simulink model "building_HVAC_V00_027_AI_2019b"  (R2021b)
settings: Solver=ode3  StartTime=1425600  StopTime=1429297  FixedStep=0.1  RelTol=1e-3
model workspace (MAT data in the model file):
  A = 0
  pystep = 1
values from neighbouring files (symbols this model uses):
  Air_Cp = [1007 1007 1006 1006 1006 1006 1006 1006 1006 1006 1007 1007 ... (21 elements, 21x1)]    [data_07.mat]    (also in data_08.mat)
  Air_density = [1.783 1.582 1.422 1.367 1.341 1.316 1.292 1.268 1.246 1.225 1.204 1.184 ... (32 elements, 32x1)]    [data_07.mat]    (also in data_08.mat)
  Air_dynamic_viscosity_PaS = [1.318e-05 1.456e-05 1.588e-05 1.64e-05 1.665e-05 1.69e-05 1.715e-05 1.74e-05 1.764e-05 1.789e-05 1.813e-05 1.837e-05 ... (32 elements, 32x1)]    [data_07.mat]    (also in data_08.mat)
  Air_enthalpy = [325420 335490 345550 355620 365680 375730 385790 395850 405910 415970 426040 436110 ... (21 elements, 21x1)]    [data_07.mat]    (also in data_08.mat)
  Air_prandtl_number = [0.734 0.72 0.711 0.707 0.705 0.701 0.699 0.698 0.699 0.702]    [data_07.mat]    (also in data_08.mat)
  Air_Temp_for_Cp = [200 210 220 230 240 250 260 270 280 290 300 310 ... (21 elements, 21x1)]    [data_07.mat]    (also in data_08.mat)
  Air_Temp_for_density = [-75 -50 -25 -15 -10 -5 0 5 10 15 20 25 ... (32 elements, 32x1)]    [data_07.mat]    (also in data_08.mat)
  Air_Temp_for_dynamic_viscosity = [-75 -50 -25 -15 -10 -5 0 5 10 15 20 25 ... (32 elements, 32x1)]    [data_07.mat]    (also in data_08.mat)
  Air_Temp_for_enthalpy = [200 210 220 230 240 250 260 270 280 290 300 310 ... (21 elements, 21x1)]    [data_07.mat]    (also in data_08.mat)
  Air_Temp_for_prandtl_number = [-100 -50 0 25 50 100 150 200 250 300]    [data_07.mat]    (also in data_08.mat)
  Air_Temp_for_thermal_conductivity = [-190 -150 -100 -75 -50 -25 -15 -10 -5 0 5 10 ... (35 elements, 35x1)]    [data_07.mat]    (also in data_08.mat)
  Air_thermal_conductivity = [0.00782 0.01169 0.0162 0.01834 0.02041 0.02241 0.0232 0.02359 0.02397 0.02436 0.02474 0.02512 ... (35 elements, 35x1)]    [data_07.mat]    (also in data_08.mat)
  Ambient_Solar_heat_Seoul_20200701_to_20200731 = [0 0 0 0 0 0 2.777777778 38.88888889 72.22222222 97.22222222 333.3333333 263.8888889 ... (745 elements, 745x1)]    [data_07.mat]    (also in data_08.mat)
  Ambient_Solar_heat_Seoul_20200701_to_20210630 = [0 0 0 0 0 2.777777778 38.88888889 72.22222222 97.22222222 333.3333333 263.8888889 152.7777778 ... (8736 elements, 8736x1)]    [data_07.mat]    (also in data_08.mat)
  Ambient_Solar_heat_Seoul_20200801_to_20200831 = [0 0 0 0 0 0 2.777777778 11.11111111 38.88888889 63.88888889 127.7777778 258.3333333 ... (745 elements, 745x1)]    [data_07.mat]    (also in data_08.mat)
  Ambient_Solar_heat_Seoul_20200901_to_20200930 = [0 0 0 0 0 0 0 22.22222222 108.3333333 141.6666667 211.1111111 386.1111111 ... (721 elements, 721x1)]    [data_07.mat]    (also in data_08.mat)
  Ambient_Temp_Seoul_20200701_to_20200731 = [18.8 18.8 18.7 18.4 18.2 18.2 18.3 18.5 19.1 19.6 21.2 21.6 ... (745 elements, 745x1)]    [data_07.mat]    (also in data_08.mat)
  Ambient_Temp_Seoul_20200701_to_20210630 = [18.8 18.7 18.4 18.2 18.2 18.3 18.5 19.1 19.6 21.2 21.6 21.7 ... (8736 elements, 8736x1)]    [data_07.mat]    (also in data_08.mat)
  Ambient_Temp_Seoul_20200801_to_20200831 = [25 24.6 24.6 24.7 24.7 24.5 24.3 24.3 24.6 25 25.7 26.8 ... (745 elements, 745x1)]    [data_07.mat]    (also in data_08.mat)
  Ambient_Temp_Seoul_20200901_to_20200930 = [26.2 25.8 25.5 24.9 24.5 24.3 24 23.9 24.4 24.8 25.7 26.6 ... (721 elements, 721x1)]    [data_07.mat]    (also in data_08.mat)
  Ambient_Time_Seoul_20200701_to_20200731 = [0 3600 7200 10800 14400 18000 21600 25200 28800 32400 36000 39600 ... (745 elements, 745x1)]    [data_07.mat]    (also in data_08.mat)
  Ambient_Time_Seoul_20200701_to_20210630 = [0 3600 7200 10800 14400 18000 21600 25200 28800 32400 36000 39600 ... (8736 elements, 8736x1)]    [data_07.mat]    (also in data_08.mat)
  Ambient_Time_Seoul_20200901_to_20200930 = [0 3600 7200 10800 14400 18000 21600 25200 28800 32400 36000 39600 ... (721 elements, 721x1)]    [data_07.mat]    (also in data_08.mat)
  Ambient_Water_Vapor_Pressure_Seoul_20200701_to_20200731 = [18.4 18.8 18.6 18.2 17.9 17.7 18.6 18.6 18.5 19.1 19.9 19.5 ... (745 elements, 745x1)]    [data_07.mat]    (also in data_08.mat)
  Ambient_Water_Vapor_Pressure_Seoul_20200701_to_20210630 = [18.8 18.6 18.2 17.9 17.7 18.6 18.6 18.5 19.1 19.9 19.5 19.4 ... (8736 elements, 8736x1)]    [data_07.mat]    (also in data_08.mat)
  Ambient_Water_Vapor_Pressure_Seoul_20200801_to_20200831 = [28.4 27.7 28.1 28.8 29.1 28.8 28.8 29.1 29.7 30 31.3 29.8 ... (745 elements, 745x1)]    [data_07.mat]    (also in data_08.mat)
  Ambient_Water_Vapor_Pressure_Seoul_20200901_to_20200930 = [26.1 25.8 25.6 24.7 24 24.3 22.9 23.1 23.1 22.8 24 24.3 ... (721 elements, 721x1)]    [data_07.mat]    (also in data_08.mat)
  Ambient_wind_speed_Seoul_20200701_to_20200731 = [3.7 3 3 2.3 1.2 1.5 3.1 1.4 1 1.4 2.5 2.1 ... (745 elements, 745x1)]    [data_07.mat]    (also in data_08.mat)
  Ambient_wind_speed_Seoul_20200701_to_20210630 = [3 3 2.3 1.2 1.5 3.1 1.4 1 1.4 2.5 2.1 2 ... (8736 elements, 8736x1)]    [data_07.mat]    (also in data_08.mat)
  Ambient_wind_speed_Seoul_20200801_to_20200831 = [3.4 0.5 0.5 1.2 0.8 1.3 1.8 1.4 1.2 1.1 1.8 3.4 ... (745 elements, 745x1)]    [data_07.mat]    (also in data_08.mat)
  Ambient_wind_speed_Seoul_20200901_to_20200930 = [2.3 2.2 2.5 2.6 2.4 2.1 1.7 2.7 2.6 2.5 1.5 1.8 ... (721 elements, 721x1)]    [data_07.mat]    (also in data_08.mat)
  init_time = start_time +60    [SIMULINK_RUn.m]    (also in data_07.mat = 0; data_08.mat = 1425660)
  Initial_Temp = 273 + 28    (= 301)    [SIMULINK_RUn.m]    (also in data_07.mat = 285; data_08.mat = 302)
  Shadow_20200701_to_20210630 = [285 300 315 330 345 360 15 30 45 60 75 90 ... (8736 elements, 8736x1)]    [data_07.mat]    (also in data_08.mat)
  start_time = 12 * 3600 + da * day_to_sec    [SIMULINK_RUn.m]    (also in data_07.mat = 0; data_08.mat = 1425600)
  Under_30cm_ground_Temp_Seoul_20200701_to_20200731 = [22.6 22.6 22.5 22.5 22.4 22.3 22.3 22.2 22.1 22.1 22 22 ... (745 elements, 745x1)]    [data_07.mat]    (also in data_08.mat)
  Under_30cm_ground_Temp_Seoul_20200701_to_20210630 = [22.6 22.5 22.5 22.4 22.3 22.3 22.2 22.1 22.1 22 22 22 ... (8736 elements, 8736x1)]    [data_07.mat]    (also in data_08.mat)
  Under_30cm_ground_Temp_Seoul_20200801_to_20200831 = [25.6 25.6 25.6 25.5 25.5 25.5 25.4 25.4 25.3 25.3 25.3 25.2 ... (745 elements, 745x1)]    [data_07.mat]    (also in data_08.mat)
  Under_30cm_ground_Temp_Seoul_20200901_to_20200930 = [27.4 27.4 27.4 27.4 27.3 27.3 27.3 27.2 27.2 27.1 27 27 ... (721 elements, 721x1)]    [data_07.mat]    (also in data_08.mat)
  water_saturation_enthalpy_latent = [2500899.39 2498955.8 2496540.3 2494128 2491818 2489411 2487006 2484604 2482303 2479905 2477508 2475213 ... (64 elements, 64x1)]    [data_07.mat]    (also in data_08.mat)
  water_saturation_enthalpy_vapor = [2500900 2502500 2504300 2506100 2508000 2509800 2511600 2513400 2515300 2517100 2518900 2520800 ... (64 elements, 64x1)]    [data_07.mat]    (also in data_08.mat)
  water_saturation_pressure = [611.65 650.03 698.46 750.07 805.02 863.5 925.7 991.83 1062.2 1136.8 1216 1300 ... (64 elements, 64x1)]    [data_07.mat]    (also in data_08.mat)
  water_Temp_for_saturation_enthalpy_latent = [273.16 274 275 276 277 278 279 280 281 282 283 284 ... (64 elements, 64x1)]    [data_07.mat]    (also in data_08.mat)
  water_Temp_for_saturation_enthalpy_vapor = [273.16 274 275 276 277 278 279 280 281 282 283 284 ... (64 elements, 64x1)]    [data_07.mat]    (also in data_08.mat)
  water_Temp_for_saturation_pressure = [273.16 274 275 276 277 278 279 280 281 282 283 284 ... (64 elements, 64x1)]    [data_07.mat]    (also in data_08.mat)
undefined symbols (not defined in the file or in its folder): DiscIntNeverNeededParam
libraries: fuzblock x1
(part 3 of 3)

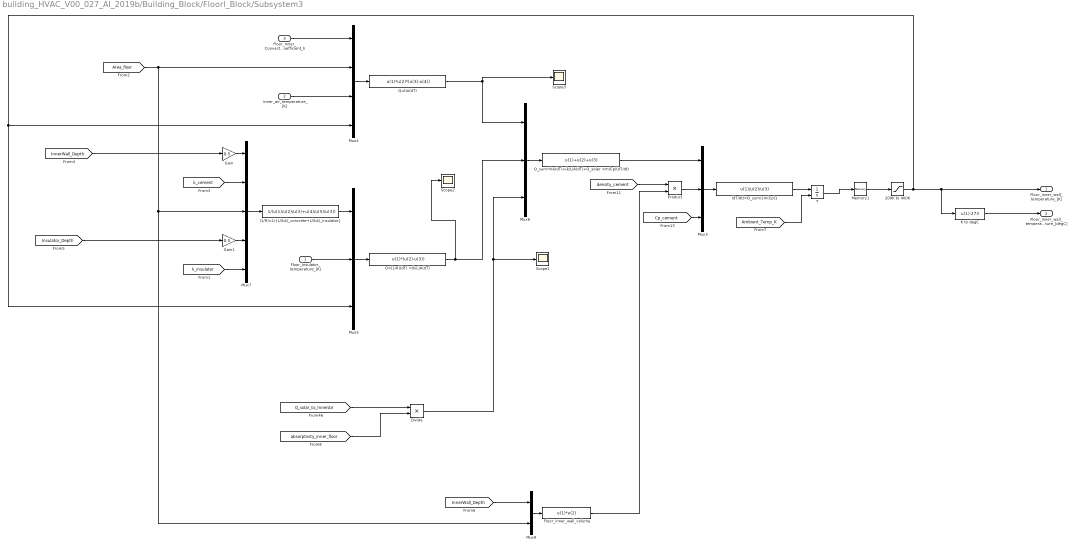
== system building_HVAC_V00_027_AI_2019b/Building_Block/Floorl_Block/Subsystem3 ==
  Floor_Insulator_temperature_[K] : Inport
  Inner_air_temperature_[K] : Inport  Port=2
  Floor_Inner_Convective_coefficient_h : Inport  Port=3
  "(1/R)=1/{L/(kA)_concrete+L/(kA)_insulator}" : Fcn  Expr=1/(u(1)/u(2)/u(3)+u(4)/u(5)/u(3))
  "(dT/dt)=Q_sum/{m(Cp)}" : Fcn  Expr=u(1)/u(2)/u(3)
  200K to 400K : Saturate  UpperLimit=400  LowerLimit=200
  Divide : Product  Inputs=**
  Floor_inner_wall_volume : Fcn  Expr=u(1)*u(2)
  Gain : Gain  Gain=0.5
  Gain1 : Gain  Gain=0.5
  K to degC : Fcn  Expr=u(1)-273
  Memory1 : Memory  InitialCondition=300-5-3  InheritSampleTime=on
  Mux3 : Mux  Inputs=3
  Mux4 : Mux
  Mux5 : Mux  Inputs=3
  Mux6 : Mux  Inputs=3
  Mux7 : Mux  Inputs=5
  Mux9 : Mux  Inputs=2
  Product : Product
  Q=(1/R)(dT) =(k/L)A(dT) : Fcn  Expr=u(1)*(u(2)-u(3))
  Q=hA(dT) : Fcn  Expr=u(1)*u(2)*(u(3)-u(4))
  Q_sum=hA(dT)+(k/L)A(dT)+Q_solar =m(Cp)(dT/dt) : Fcn  Expr=u(1)+u(2)+u(3)
  Scope1 : Scope
  Scope2 : Scope
  Scope3 : Scope
  T : Integrator  InitialConditionSource=external
  Floor_inner_wall_temperature_[K] : Outport
  Floor_inner_wall_temperature_[degC] : Outport  Port=2
  wires:
  K to degC/1 -> Floor_inner_wall_temperature_[degC]/1
  Floor_inner_wall_volume/1 -> Product/2
  [k_insulator] -> Mux7/5
  Gain1/1 -> Mux7/4
  Floor_Insulator_temperature_[K]/1 -> Mux5/2
  Q_sum=hA(dT)+(k/L)A(dT)+Q_solar =m(Cp)(dT/dt)/1 -> Mux3/1
  [k_cement] -> Mux7/2
  Mux7/1 -> "(1/R)=1/{L/(kA)_concrete+L/(kA)_insulator}"/1
  Q=hA(dT)/1 -> Mux6/1, Scope3/1
  "(1/R)=1/{L/(kA)_concrete+L/(kA)_insulator}"/1 -> Mux5/1
  Gain/1 -> Mux7/1
  Memory1/1 -> 200K to 400K/1
  Q=(1/R)(dT) =(k/L)A(dT)/1 -> Scope2/1, Mux6/2
  Mux4/1 -> Q=hA(dT)/1
  Mux5/1 -> Q=(1/R)(dT) =(k/L)A(dT)/1
  200K to 400K/1 -> Mux5/3, Mux4/4, Floor_inner_wall_temperature_[K]/1, K to degC/1
  T/1 -> Memory1/1
  Inner_air_temperature_[K]/1 -> Mux4/3
  [Area_floor] -> Mux9/2, Mux7/3, Mux4/2
  Product/1 -> Mux3/2
  [Cp_cement] -> Mux3/3
  "(dT/dt)=Q_sum/{m(Cp)}"/1 -> T/1
  Mux9/1 -> Floor_inner_wall_volume/1
  [density_cement] -> Product/1
  Mux3/1 -> "(dT/dt)=Q_sum/{m(Cp)}"/1
  Floor_Inner_Convective_coefficient_h/1 -> Mux4/1
  Mux6/1 -> Q_sum=hA(dT)+(k/L)A(dT)+Q_solar =m(Cp)(dT/dt)/1
  [Ambient_Temp_K] -> T/2
  [Q_solar_to_InnerAir] -> Divide/1
  [absorptivity_inner_floor] -> Divide/2
  [InnerWall_Depth] -> Gain/1
  [Insulator_Depth] -> Gain1/1
  Divide/1 -> Scope1/1, Mux6/3
  [InnerWall_Depth] -> Mux9/1

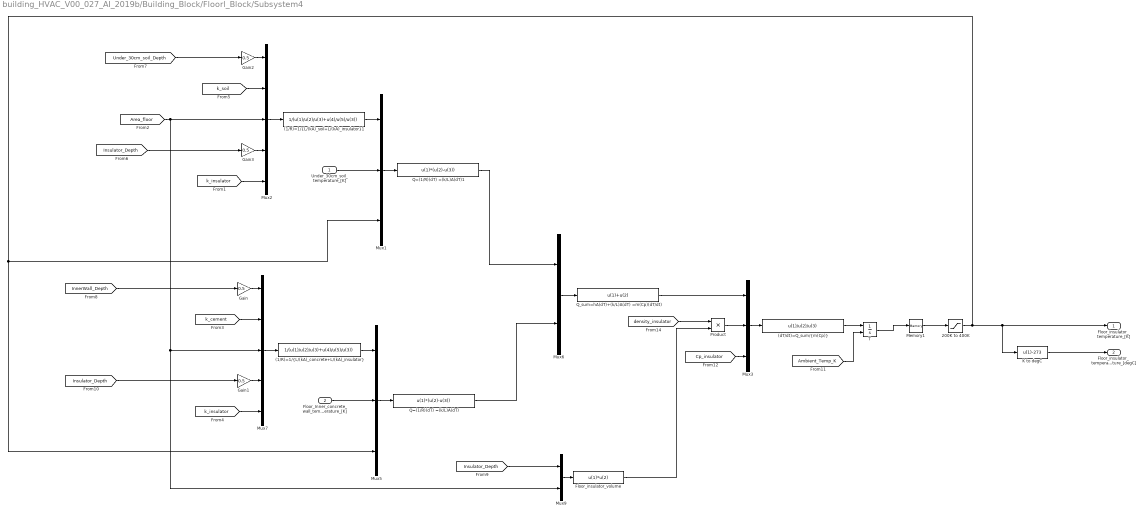
== system building_HVAC_V00_027_AI_2019b/Building_Block/Floorl_Block/Subsystem4 ==
  Under_30cm_soil_temperature_[K] : Inport
  Floor_Inner_concrete_wall_temperature_[K] : Inport  Port=2
  "(1/R)=1/{L/(kA)_concrete+L/(kA)_insulator}" : Fcn  Expr=1/(u(1)/u(2)/u(3)+u(4)/u(5)/u(3))
  "(1/R)=1/{L/(kA)_soil+L/(kA)_insulator}1" : Fcn  Expr=1/(u(1)/u(2)/u(3)+u(4)/u(5)/u(3))
  "(dT/dt)=Q_sum/{m(Cp)}" : Fcn  Expr=u(1)/u(2)/u(3)
  200K to 400K : Saturate  UpperLimit=400  LowerLimit=200
  Floor_insulator_volume : Fcn  Expr=u(1)*u(2)
  Gain{,1..3} (4 alike) : Gain  Gain=0.5
  K to degC : Fcn  Expr=u(1)-273
  Memory1 : Memory  InitialCondition=300  InheritSampleTime=on
  Mux1 : Mux  Inputs=3
  Mux2 : Mux  Inputs=5
  Mux3 : Mux  Inputs=3
  Mux5 : Mux  Inputs=3
  Mux6 : Mux  Inputs=2
  Mux7 : Mux  Inputs=5
  Mux9 : Mux  Inputs=2
  Product : Product
  Q=(1/R)(dT) =(k/L)A(dT) : Fcn  Expr=u(1)*(u(2)-u(3))
  Q=(1/R)(dT) =(k/L)A(dT)1 : Fcn  Expr=u(1)*(u(2)-u(3))
  Q_sum=hA(dT)+(k/L)A(dT) =m(Cp)(dT/dt) : Fcn  Expr=u(1)+u(2)
  T : Integrator  InitialConditionSource=external
  Floor_insulator_temperature_[K] : Outport
  Floor_insulator_temperature_[degC] : Outport  Port=2
  wires:
  Mux6/1 -> Q_sum=hA(dT)+(k/L)A(dT) =m(Cp)(dT/dt)/1
  Mux3/1 -> "(dT/dt)=Q_sum/{m(Cp)}"/1
  [density_insulator] -> Product/1
  Mux9/1 -> Floor_insulator_volume/1
  "(dT/dt)=Q_sum/{m(Cp)}"/1 -> T/1
  [Cp_insulator] -> Mux3/3
  Product/1 -> Mux3/2
  [Area_floor] -> Mux9/2, Mux7/3, Mux2/3
  T/1 -> Memory1/1
  200K to 400K/1 -> K to degC/1, Floor_insulator_temperature_[K]/1, Mux1/3, Mux5/3
  Mux5/1 -> Q=(1/R)(dT) =(k/L)A(dT)/1
  Q=(1/R)(dT) =(k/L)A(dT)/1 -> Mux6/2
  Memory1/1 -> 200K to 400K/1
  Gain/1 -> Mux7/1
  "(1/R)=1/{L/(kA)_concrete+L/(kA)_insulator}"/1 -> Mux5/1
  Q=(1/R)(dT) =(k/L)A(dT)1/1 -> Mux6/1
  Mux7/1 -> "(1/R)=1/{L/(kA)_concrete+L/(kA)_insulator}"/1
  [k_cement] -> Mux7/2
  Q_sum=hA(dT)+(k/L)A(dT) =m(Cp)(dT/dt)/1 -> Mux3/1
  Floor_Inner_concrete_wall_temperature_[K]/1 -> Mux5/2
  Gain1/1 -> Mux7/4
  [k_insulator] -> Mux7/5
  Floor_insulator_volume/1 -> Product/2
  K to degC/1 -> Floor_insulator_temperature_[degC]/1
  [k_insulator] -> Mux2/5
  "(1/R)=1/{L/(kA)_soil+L/(kA)_insulator}1"/1 -> Mux1/1
  Gain2/1 -> Mux2/1
  [k_soil] -> Mux2/2
  Mux1/1 -> Q=(1/R)(dT) =(k/L)A(dT)1/1
  Under_30cm_soil_temperature_[K]/1 -> Mux1/2
  Mux2/1 -> "(1/R)=1/{L/(kA)_soil+L/(kA)_insulator}1"/1
  Gain3/1 -> Mux2/4
  [Ambient_Temp_K] -> T/2
  [Under_30cm_soil_Depth] -> Gain2/1
  [Insulator_Depth] -> Gain3/1
  [InnerWall_Depth] -> Gain/1
  [Insulator_Depth] -> Gain1/1
  [Insulator_Depth] -> Mux9/1

== system building_HVAC_V00_027_AI_2019b/Building_Block/North_Wall_Block/Subsystem1 ==
  North_inner_concrete_wall_temperature_[K] : Inport
  Inner_air_temperature_[K] : Inport  Port=2
  North_Inner_Convective_coefficient_h : Inport  Port=3
  -1000000 to 1000000 : Saturate  UpperLimit=1000000  LowerLimit=-1000000
  Memory : Memory  InheritSampleTime=on
  Mux4 : Mux
  Q=hA(dT) : Fcn  Expr=u(1)*u(2)*(u(3)-u(4))
  Q_North_InnerWall_to_InnerAir_[W] : Outport
  wires:
  Memory/1 -> -1000000 to 1000000/1
  Q=hA(dT)/1 -> Memory/1
  Mux4/1 -> Q=hA(dT)/1
  -1000000 to 1000000/1 -> Q_North_InnerWall_to_InnerAir_[W]/1
  North_inner_concrete_wall_temperature_[K]/1 -> Mux4/3
  [Area_North] -> Mux4/2
  North_Inner_Convective_coefficient_h/1 -> Mux4/1
  Inner_air_temperature_[K]/1 -> Mux4/4

== system building_HVAC_V00_027_AI_2019b/Building_Block/North_Wall_Block/Subsystem2 ==
  Ambient_temperature_[K] : Inport
  North_Insulator_temperature_[K] : Inport  Port=2
  North_Out_Convective_coefficient_h : Inport  Port=3
  "(1/R)=1/{L/(kA)_concrete+L/(kA)_insulator}" : Fcn  Expr=1/(u(1)/u(2)/u(3)+u(4)/u(5)/u(3))
  "(dT/dt)=Q_sum/{m(Cp)}" : Fcn  Expr=u(1)/u(2)/u(3)
  200K to 800K : Saturate  UpperLimit=800  LowerLimit=200
  Divide : Product  Inputs=***
  Gain : Gain  Gain=0.5
  Gain1 : Gain  Gain=0.5
  K to degC : Fcn  Expr=u(1)-273
  Memory1 : Memory  InitialCondition=300  InheritSampleTime=on
  Mux3 : Mux  Inputs=3
  Mux4 : Mux
  Mux5 : Mux  Inputs=3
  Mux6 : Mux  Inputs=3
  Mux7 : Mux  Inputs=5
  Mux9 : Mux  Inputs=2
  North_wall_volume : Fcn  Expr=u(1)*u(2)
  Product : Product
  Q=(1/R)(dT) =(k/L)A(dT) : Fcn  Expr=u(1)*(u(2)-u(3))
  Q=hA(dT) : Fcn  Expr=u(1)*u(2)*(u(3)-u(4))
  Q_sum=hA(dT)+(k/L)A(dT)+Q_solar =m(Cp)(dT/dt) : Fcn  Expr=u(1)+u(2)+u(3)
  T : Integrator  InitialConditionSource=external
  North_outer_concrete_wall_temperature_[K] : Outport
  North_outer_concrete_wall_temperature_[degC] : Outport  Port=2
  wires:
  [absoptivity_wall] -> Divide/2
  [solar_heat_flux] -> Divide/3
  Divide/1 -> Mux6/3
  [Area_North] -> Mux4/2, Mux7/3, Divide/1, Mux9/2
  K to degC/1 -> North_outer_concrete_wall_temperature_[degC]/1
  North_wall_volume/1 -> Product/2
  [k_insulator] -> Mux7/5
  Gain1/1 -> Mux7/4
  North_Insulator_temperature_[K]/1 -> Mux5/2
  Q_sum=hA(dT)+(k/L)A(dT)+Q_solar =m(Cp)(dT/dt)/1 -> Mux3/1
  [k_cement] -> Mux7/2
  Mux7/1 -> "(1/R)=1/{L/(kA)_concrete+L/(kA)_insulator}"/1
  Q=hA(dT)/1 -> Mux6/1
  "(1/R)=1/{L/(kA)_concrete+L/(kA)_insulator}"/1 -> Mux5/1
  Gain/1 -> Mux7/1
  [Insulator_Depth] -> Gain1/1
  Memory1/1 -> 200K to 800K/1
  Q=(1/R)(dT) =(k/L)A(dT)/1 -> Mux6/2
  Mux4/1 -> Q=hA(dT)/1
  Mux5/1 -> Q=(1/R)(dT) =(k/L)A(dT)/1
  200K to 800K/1 -> Mux5/3, Mux4/4, North_outer_concrete_wall_temperature_[K]/1, K to degC/1
  T/1 -> Memory1/1
  [OuterWall_Depth] -> Gain/1
  Ambient_temperature_[K]/1 -> Mux4/3
  [OuterWall_Depth] -> Mux9/1
  Product/1 -> Mux3/2
  [Cp_cement] -> Mux3/3
  "(dT/dt)=Q_sum/{m(Cp)}"/1 -> T/1
  Mux9/1 -> North_wall_volume/1
  [density_cement] -> Product/1
  Mux3/1 -> "(dT/dt)=Q_sum/{m(Cp)}"/1
  North_Out_Convective_coefficient_h/1 -> Mux4/1
  Mux6/1 -> Q_sum=hA(dT)+(k/L)A(dT)+Q_solar =m(Cp)(dT/dt)/1
  [Ambient_Temp_K] -> T/2

== system building_HVAC_V00_027_AI_2019b/Building_Block/North_Wall_Block/Subsystem3 ==
  North_Insulator_temperature_[K] : Inport
  Inner_air_temperature_[K] : Inport  Port=2
  North_Inner_Convective_coefficient_h : Inport  Port=3
  "(1/R)=1/{L/(kA)_concrete+L/(kA)_insulator}" : Fcn  Expr=1/(u(1)/u(2)/u(3)+u(4)/u(5)/u(3))
  "(dT/dt)=Q_sum/{m(Cp)}" : Fcn  Expr=u(1)/u(2)/u(3)
  200K to 400K : Saturate  UpperLimit=400  LowerLimit=200
  Divide : Product  Inputs=**
  Gain : Gain  Gain=0.5
  Gain1 : Gain  Gain=0.5
  K to degC : Fcn  Expr=u(1)-273
  Memory1 : Memory  InitialCondition=300  InheritSampleTime=on
  Mux3 : Mux  Inputs=3
  Mux4 : Mux
  Mux5 : Mux  Inputs=3
  Mux6 : Mux  Inputs=3
  Mux7 : Mux  Inputs=5
  Mux9 : Mux  Inputs=2
  North_wall_volume : Fcn  Expr=u(1)*u(2)
  Product : Product
  Q=(1/R)(dT) =(k/L)A(dT) : Fcn  Expr=u(1)*(u(2)-u(3))
  Q=hA(dT) : Fcn  Expr=u(1)*u(2)*(u(3)-u(4))
  Q_sum=hA(dT)+(k/L)A(dT)+Q_solar =m(Cp)(dT/dt) : Fcn  Expr=u(1)+u(2)
  T : Integrator  InitialConditionSource=external
  North_inner_concrete_wall_temperature_[K] : Outport
  North_inner_concrete_wall_temperature_[degC] : Outport  Port=2
  wires:
  Mux6/1 -> Q_sum=hA(dT)+(k/L)A(dT)+Q_solar =m(Cp)(dT/dt)/1
  North_Inner_Convective_coefficient_h/1 -> Mux4/1
  Mux3/1 -> "(dT/dt)=Q_sum/{m(Cp)}"/1
  [density_cement] -> Product/1
  Mux9/1 -> North_wall_volume/1
  "(dT/dt)=Q_sum/{m(Cp)}"/1 -> T/1
  [Cp_cement] -> Mux3/3
  Product/1 -> Mux3/2
  [InnerWall_Depth] -> Mux9/1
  [Area_North] -> Mux4/2, Mux7/3, Mux9/2
  Inner_air_temperature_[K]/1 -> Mux4/3
  [InnerWall_Depth] -> Gain/1
  T/1 -> Memory1/1
  200K to 400K/1 -> K to degC/1, North_inner_concrete_wall_temperature_[K]/1, Mux4/4, Mux5/3
  Mux5/1 -> Q=(1/R)(dT) =(k/L)A(dT)/1
  Mux4/1 -> Q=hA(dT)/1
  Q=(1/R)(dT) =(k/L)A(dT)/1 -> Mux6/2
  Memory1/1 -> 200K to 400K/1
  [Insulator_Depth] -> Gain1/1
  Gain/1 -> Mux7/1
  "(1/R)=1/{L/(kA)_concrete+L/(kA)_insulator}"/1 -> Mux5/1
  Q=hA(dT)/1 -> Mux6/1
  Mux7/1 -> "(1/R)=1/{L/(kA)_concrete+L/(kA)_insulator}"/1
  [k_cement] -> Mux7/2
  Q_sum=hA(dT)+(k/L)A(dT)+Q_solar =m(Cp)(dT/dt)/1 -> Mux3/1
  North_Insulator_temperature_[K]/1 -> Mux5/2
  Gain1/1 -> Mux7/4
  [k_insulator] -> Mux7/5
  North_wall_volume/1 -> Product/2
  K to degC/1 -> North_inner_concrete_wall_temperature_[degC]/1
  [Ambient_Temp_K] -> T/2
  [absorptivity_inner_wall_North] -> Divide/2
  [Q_solar_to_InnerAir] -> Divide/1
  Divide/1 -> Mux6/3

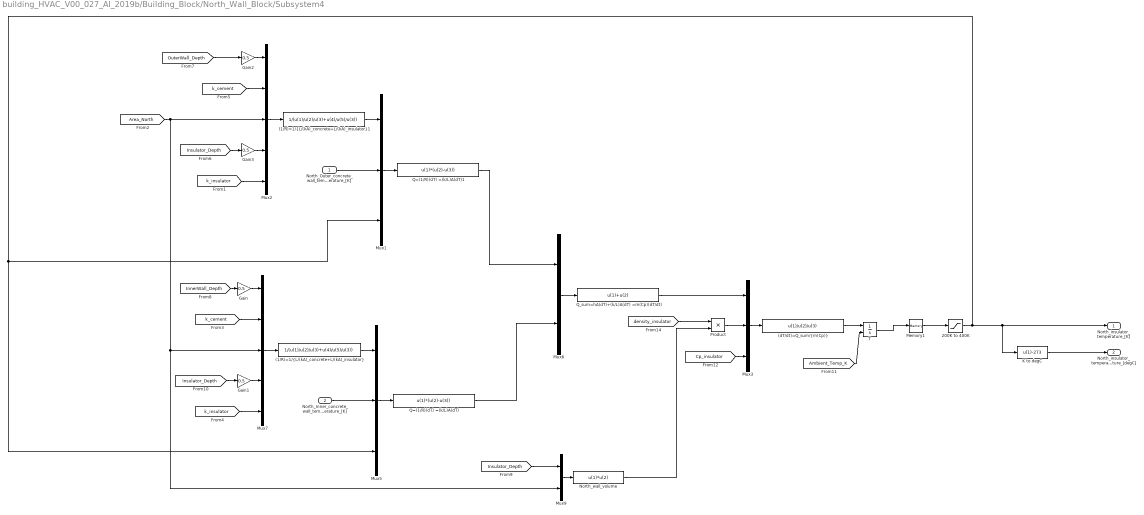
== system building_HVAC_V00_027_AI_2019b/Building_Block/North_Wall_Block/Subsystem4 ==
  North_Outer_concrete_wall_temperature_[K] : Inport
  North_Inner_concrete_wall_temperature_[K] : Inport  Port=2
  "(1/R)=1/{L/(kA)_concrete+L/(kA)_insulator}" : Fcn  Expr=1/(u(1)/u(2)/u(3)+u(4)/u(5)/u(3))
  "(1/R)=1/{L/(kA)_concrete+L/(kA)_insulator}1" : Fcn  Expr=1/(u(1)/u(2)/u(3)+u(4)/u(5)/u(3))
  "(dT/dt)=Q_sum/{m(Cp)}" : Fcn  Expr=u(1)/u(2)/u(3)
  200K to 400K : Saturate  UpperLimit=400  LowerLimit=200
  Gain{,1..3} (4 alike) : Gain  Gain=0.5
  K to degC : Fcn  Expr=u(1)-273
  Memory1 : Memory  InitialCondition=300  InheritSampleTime=on
  Mux1 : Mux  Inputs=3
  Mux2 : Mux  Inputs=5
  Mux3 : Mux  Inputs=3
  Mux5 : Mux  Inputs=3
  Mux6 : Mux  Inputs=2
  Mux7 : Mux  Inputs=5
  Mux9 : Mux  Inputs=2
  North_wall_volume : Fcn  Expr=u(1)*u(2)
  Product : Product
  Q=(1/R)(dT) =(k/L)A(dT) : Fcn  Expr=u(1)*(u(2)-u(3))
  Q=(1/R)(dT) =(k/L)A(dT)1 : Fcn  Expr=u(1)*(u(2)-u(3))
  Q_sum=hA(dT)+(k/L)A(dT) =m(Cp)(dT/dt) : Fcn  Expr=u(1)+u(2)
  T : Integrator  InitialConditionSource=external
  North_insulator_temperature_[K] : Outport
  North_insulator_temperature_[degC] : Outport  Port=2
  wires:
  [OuterWall_Depth] -> Gain2/1
  Gain3/1 -> Mux2/4
  Mux2/1 -> "(1/R)=1/{L/(kA)_concrete+L/(kA)_insulator}1"/1
  North_Outer_concrete_wall_temperature_[K]/1 -> Mux1/2
  Mux1/1 -> Q=(1/R)(dT) =(k/L)A(dT)1/1
  [Insulator_Depth] -> Gain3/1
  [k_cement] -> Mux2/2
  Gain2/1 -> Mux2/1
  "(1/R)=1/{L/(kA)_concrete+L/(kA)_insulator}1"/1 -> Mux1/1
  [k_insulator] -> Mux2/5
  K to degC/1 -> North_insulator_temperature_[degC]/1
  North_wall_volume/1 -> Product/2
  [k_insulator] -> Mux7/5
  Gain1/1 -> Mux7/4
  North_Inner_concrete_wall_temperature_[K]/1 -> Mux5/2
  Q_sum=hA(dT)+(k/L)A(dT) =m(Cp)(dT/dt)/1 -> Mux3/1
  [k_cement] -> Mux7/2
  Mux7/1 -> "(1/R)=1/{L/(kA)_concrete+L/(kA)_insulator}"/1
  Q=(1/R)(dT) =(k/L)A(dT)1/1 -> Mux6/1
  "(1/R)=1/{L/(kA)_concrete+L/(kA)_insulator}"/1 -> Mux5/1
  Gain/1 -> Mux7/1
  [Insulator_Depth] -> Gain1/1
  Memory1/1 -> 200K to 400K/1
  Q=(1/R)(dT) =(k/L)A(dT)/1 -> Mux6/2
  Mux5/1 -> Q=(1/R)(dT) =(k/L)A(dT)/1
  200K to 400K/1 -> Mux5/3, Mux1/3, North_insulator_temperature_[K]/1, K to degC/1
  T/1 -> Memory1/1
  [InnerWall_Depth] -> Gain/1
  [Area_North] -> Mux2/3, Mux7/3, Mux9/2
  [Insulator_Depth] -> Mux9/1
  Product/1 -> Mux3/2
  [Cp_insulator] -> Mux3/3
  "(dT/dt)=Q_sum/{m(Cp)}"/1 -> T/1
  Mux9/1 -> North_wall_volume/1
  [density_insulator] -> Product/1
  Mux3/1 -> "(dT/dt)=Q_sum/{m(Cp)}"/1
  Mux6/1 -> Q_sum=hA(dT)+(k/L)A(dT) =m(Cp)(dT/dt)/1
  [Ambient_Temp_K] -> T/2

== system building_HVAC_V00_027_AI_2019b/Building_Block/South_Wall_Block/Subsystem1 ==
  South_inner_concrete_wall_temperature_[K] : Inport
  Inner_air_temperature_[K] : Inport  Port=2
  South_Inner_Convective_coefficient_h : Inport  Port=3
  -1000000 to 1000000 : Saturate  UpperLimit=1000000  LowerLimit=-1000000
  Memory : Memory  InheritSampleTime=on
  Mux4 : Mux
  Q=hA(dT) : Fcn  Expr=u(1)*u(2)*(u(3)-u(4))
  Q_South_InnerWall_to_InnerAir_[W] : Outport
  wires:
  South_Inner_Convective_coefficient_h/1 -> Mux4/1
  [Area_South] -> Mux4/2
  -1000000 to 1000000/1 -> Q_South_InnerWall_to_InnerAir_[W]/1
  Mux4/1 -> Q=hA(dT)/1
  Q=hA(dT)/1 -> Memory/1
  Memory/1 -> -1000000 to 1000000/1
  South_inner_concrete_wall_temperature_[K]/1 -> Mux4/3
  Inner_air_temperature_[K]/1 -> Mux4/4

== system building_HVAC_V00_027_AI_2019b/Building_Block/South_Wall_Block/Subsystem2 ==
  Ambient_temperature_[K] : Inport
  South_Insulator_temperature_[K] : Inport  Port=2
  South_Out_Convective_coefficient_h : Inport  Port=3
  "(1/R)=1/{L/(kA)_concrete+L/(kA)_insulator}" : Fcn  Expr=1/(u(1)/u(2)/u(3)+u(4)/u(5)/u(3))
  "(dT/dt)=Q_sum/{m(Cp)}" : Fcn  Expr=u(1)/u(2)/u(3)
  200K to 800K : Saturate  UpperLimit=800  LowerLimit=200
  Divide : Product  Inputs=***
  Gain : Gain  Gain=0.5
  Gain1 : Gain  Gain=0.5
  K to degC : Fcn  Expr=u(1)-273
  Memory1 : Memory  InitialCondition=300  InheritSampleTime=on
  Mux3 : Mux  Inputs=3
  Mux4 : Mux
  Mux5 : Mux  Inputs=3
  Mux6 : Mux  Inputs=3
  Mux7 : Mux  Inputs=5
  Mux9 : Mux  Inputs=2
  Product : Product
  Q=(1/R)(dT) =(k/L)A(dT) : Fcn  Expr=u(1)*(u(2)-u(3))
  Q=hA(dT) : Fcn  Expr=u(1)*u(2)*(u(3)-u(4))
  Q_sum=hA(dT)+(k/L)A(dT)+Q_solar =m(Cp)(dT/dt) : Fcn  Expr=u(1)+u(2)+u(3)
  South_wall_volume : Fcn  Expr=u(1)*u(2)
  T : Integrator  InitialConditionSource=external
  South_outer_concrete_wall_temperature_[K] : Outport
  South_outer_concrete_wall_temperature_[degC] : Outport  Port=2
  wires:
  Mux6/1 -> Q_sum=hA(dT)+(k/L)A(dT)+Q_solar =m(Cp)(dT/dt)/1
  South_Out_Convective_coefficient_h/1 -> Mux4/1
  Mux3/1 -> "(dT/dt)=Q_sum/{m(Cp)}"/1
  [density_cement] -> Product/1
  Mux9/1 -> South_wall_volume/1
  "(dT/dt)=Q_sum/{m(Cp)}"/1 -> T/1
  [Cp_cement] -> Mux3/3
  Product/1 -> Mux3/2
  [OuterWall_Depth] -> Mux9/1
  Ambient_temperature_[K]/1 -> Mux4/3
  [OuterWall_Depth] -> Gain/1
  T/1 -> Memory1/1
  200K to 800K/1 -> K to degC/1, South_outer_concrete_wall_temperature_[K]/1, Mux4/4, Mux5/3
  Mux5/1 -> Q=(1/R)(dT) =(k/L)A(dT)/1
  Mux4/1 -> Q=hA(dT)/1
  Q=(1/R)(dT) =(k/L)A(dT)/1 -> Mux6/2
  Memory1/1 -> 200K to 800K/1
  [Insulator_Depth] -> Gain1/1
  Gain/1 -> Mux7/1
  "(1/R)=1/{L/(kA)_concrete+L/(kA)_insulator}"/1 -> Mux5/1
  Q=hA(dT)/1 -> Mux6/1
  Mux7/1 -> "(1/R)=1/{L/(kA)_concrete+L/(kA)_insulator}"/1
  [k_cement] -> Mux7/2
  Q_sum=hA(dT)+(k/L)A(dT)+Q_solar =m(Cp)(dT/dt)/1 -> Mux3/1
  South_Insulator_temperature_[K]/1 -> Mux5/2
  Gain1/1 -> Mux7/4
  [k_insulator] -> Mux7/5
  South_wall_volume/1 -> Product/2
  K to degC/1 -> South_outer_concrete_wall_temperature_[degC]/1
  [Area_South] -> Mux9/2, Divide/1, Mux7/3, Mux4/2
  Divide/1 -> Mux6/3
  [solar_heat_flux] -> Divide/3
  [absoptivity_wall] -> Divide/2
  [Ambient_Temp_K] -> T/2

== system building_HVAC_V00_027_AI_2019b/Building_Block/South_Wall_Block/Subsystem3 ==
  South_Insulator_temperature_[K] : Inport
  Inner_air_temperature_[K] : Inport  Port=2
  South_Inner_Convective_coefficient_h : Inport  Port=3
  "(1/R)=1/{L/(kA)_concrete+L/(kA)_insulator}" : Fcn  Expr=1/(u(1)/u(2)/u(3)+u(4)/u(5)/u(3))
  "(dT/dt)=Q_sum/{m(Cp)}" : Fcn  Expr=u(1)/u(2)/u(3)
  200K to 400K : Saturate  UpperLimit=400  LowerLimit=200
  Divide : Product  Inputs=**
  Gain : Gain  Gain=0.5
  Gain1 : Gain  Gain=0.5
  K to degC : Fcn  Expr=u(1)-273
  Memory1 : Memory  InitialCondition=300  InheritSampleTime=on
  Mux3 : Mux  Inputs=3
  Mux4 : Mux
  Mux5 : Mux  Inputs=3
  Mux6 : Mux  Inputs=3
  Mux7 : Mux  Inputs=5
  Mux9 : Mux  Inputs=2
  Product : Product
  Q=(1/R)(dT) =(k/L)A(dT) : Fcn  Expr=u(1)*(u(2)-u(3))
  Q=hA(dT) : Fcn  Expr=u(1)*u(2)*(u(3)-u(4))
  Q_sum=hA(dT)+(k/L)A(dT)_Q_solar =m(Cp)(dT/dt) : Fcn  Expr=u(1)+u(2)
  South_wall_volume : Fcn  Expr=u(1)*u(2)
  T : Integrator  InitialConditionSource=external
  South_inner_concrete_wall_temperature_[K] : Outport
  South_inner_concrete_wall_temperature_[degC] : Outport  Port=2
  wires:
  K to degC/1 -> South_inner_concrete_wall_temperature_[degC]/1
  South_wall_volume/1 -> Product/2
  [k_insulator] -> Mux7/5
  Gain1/1 -> Mux7/4
  South_Insulator_temperature_[K]/1 -> Mux5/2
  Q_sum=hA(dT)+(k/L)A(dT)_Q_solar =m(Cp)(dT/dt)/1 -> Mux3/1
  [k_cement] -> Mux7/2
  Mux7/1 -> "(1/R)=1/{L/(kA)_concrete+L/(kA)_insulator}"/1
  Q=hA(dT)/1 -> Mux6/1
  "(1/R)=1/{L/(kA)_concrete+L/(kA)_insulator}"/1 -> Mux5/1
  Gain/1 -> Mux7/1
  [Insulator_Depth] -> Gain1/1
  Memory1/1 -> 200K to 400K/1
  Q=(1/R)(dT) =(k/L)A(dT)/1 -> Mux6/2
  Mux4/1 -> Q=hA(dT)/1
  Mux5/1 -> Q=(1/R)(dT) =(k/L)A(dT)/1
  200K to 400K/1 -> Mux5/3, Mux4/4, South_inner_concrete_wall_temperature_[K]/1, K to degC/1
  T/1 -> Memory1/1
  [InnerWall_Depth] -> Gain/1
  Inner_air_temperature_[K]/1 -> Mux4/3
  [Area_South] -> Mux9/2, Mux7/3, Mux4/2
  [InnerWall_Depth] -> Mux9/1
  Product/1 -> Mux3/2
  [Cp_cement] -> Mux3/3
  "(dT/dt)=Q_sum/{m(Cp)}"/1 -> T/1
  Mux9/1 -> South_wall_volume/1
  [density_cement] -> Product/1
  Mux3/1 -> "(dT/dt)=Q_sum/{m(Cp)}"/1
  South_Inner_Convective_coefficient_h/1 -> Mux4/1
  Mux6/1 -> Q_sum=hA(dT)+(k/L)A(dT)_Q_solar =m(Cp)(dT/dt)/1
  [Ambient_Temp_K] -> T/2
  Divide/1 -> Mux6/3
  [Q_solar_to_InnerAir] -> Divide/1
  [absorptivity_inner_wall_South] -> Divide/2

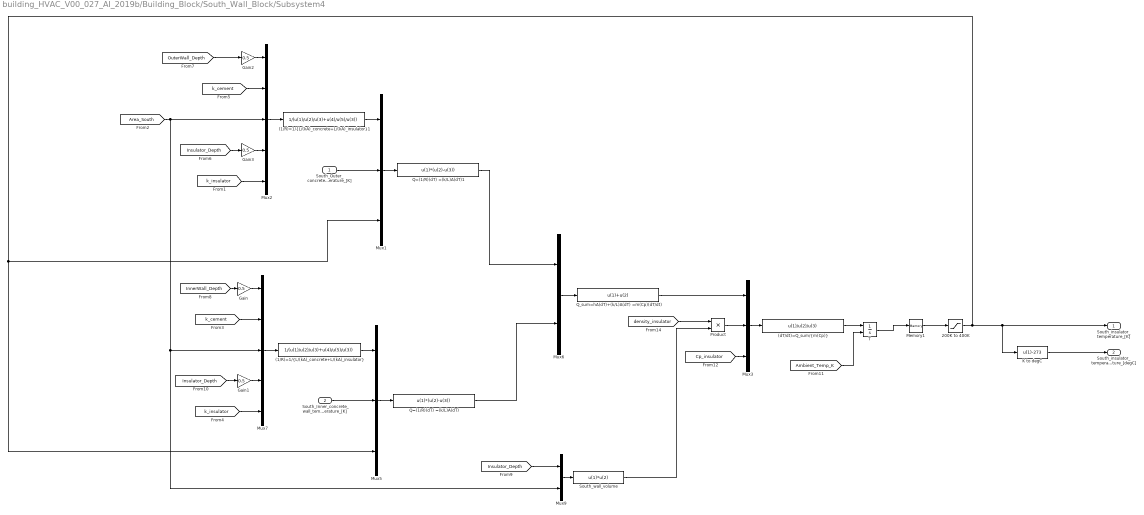
== system building_HVAC_V00_027_AI_2019b/Building_Block/South_Wall_Block/Subsystem4 ==
  South_Outer_concrete_wall_temperature_[K] : Inport
  South_Inner_concrete_wall_temperature_[K] : Inport  Port=2
  "(1/R)=1/{L/(kA)_concrete+L/(kA)_insulator}" : Fcn  Expr=1/(u(1)/u(2)/u(3)+u(4)/u(5)/u(3))
  "(1/R)=1/{L/(kA)_concrete+L/(kA)_insulator}1" : Fcn  Expr=1/(u(1)/u(2)/u(3)+u(4)/u(5)/u(3))
  "(dT/dt)=Q_sum/{m(Cp)}" : Fcn  Expr=u(1)/u(2)/u(3)
  200K to 400K : Saturate  UpperLimit=400  LowerLimit=200
  Gain{,1..3} (4 alike) : Gain  Gain=0.5
  K to degC : Fcn  Expr=u(1)-273
  Memory1 : Memory  InitialCondition=300  InheritSampleTime=on
  Mux1 : Mux  Inputs=3
  Mux2 : Mux  Inputs=5
  Mux3 : Mux  Inputs=3
  Mux5 : Mux  Inputs=3
  Mux6 : Mux  Inputs=2
  Mux7 : Mux  Inputs=5
  Mux9 : Mux  Inputs=2
  Product : Product
  Q=(1/R)(dT) =(k/L)A(dT) : Fcn  Expr=u(1)*(u(2)-u(3))
  Q=(1/R)(dT) =(k/L)A(dT)1 : Fcn  Expr=u(1)*(u(2)-u(3))
  Q_sum=hA(dT)+(k/L)A(dT) =m(Cp)(dT/dt) : Fcn  Expr=u(1)+u(2)
  South_wall_volume : Fcn  Expr=u(1)*u(2)
  T : Integrator  InitialConditionSource=external
  South_insulator_temperature_[K] : Outport
  South_insulator_temperature_[degC] : Outport  Port=2
  wires:
  Mux6/1 -> Q_sum=hA(dT)+(k/L)A(dT) =m(Cp)(dT/dt)/1
  Mux3/1 -> "(dT/dt)=Q_sum/{m(Cp)}"/1
  [density_insulator] -> Product/1
  Mux9/1 -> South_wall_volume/1
  "(dT/dt)=Q_sum/{m(Cp)}"/1 -> T/1
  [Cp_insulator] -> Mux3/3
  Product/1 -> Mux3/2
  [Insulator_Depth] -> Mux9/1
  [Area_South] -> Mux9/2, Mux7/3, Mux2/3
  [InnerWall_Depth] -> Gain/1
  T/1 -> Memory1/1
  200K to 400K/1 -> K to degC/1, South_insulator_temperature_[K]/1, Mux1/3, Mux5/3
  Mux5/1 -> Q=(1/R)(dT) =(k/L)A(dT)/1
  Q=(1/R)(dT) =(k/L)A(dT)/1 -> Mux6/2
  Memory1/1 -> 200K to 400K/1
  [Insulator_Depth] -> Gain1/1
  Gain/1 -> Mux7/1
  "(1/R)=1/{L/(kA)_concrete+L/(kA)_insulator}"/1 -> Mux5/1
  Q=(1/R)(dT) =(k/L)A(dT)1/1 -> Mux6/1
  Mux7/1 -> "(1/R)=1/{L/(kA)_concrete+L/(kA)_insulator}"/1
  [k_cement] -> Mux7/2
  Q_sum=hA(dT)+(k/L)A(dT) =m(Cp)(dT/dt)/1 -> Mux3/1
  South_Inner_concrete_wall_temperature_[K]/1 -> Mux5/2
  Gain1/1 -> Mux7/4
  [k_insulator] -> Mux7/5
  South_wall_volume/1 -> Product/2
  K to degC/1 -> South_insulator_temperature_[degC]/1
  [k_insulator] -> Mux2/5
  "(1/R)=1/{L/(kA)_concrete+L/(kA)_insulator}1"/1 -> Mux1/1
  Gain2/1 -> Mux2/1
  [k_cement] -> Mux2/2
  [Insulator_Depth] -> Gain3/1
  Mux1/1 -> Q=(1/R)(dT) =(k/L)A(dT)1/1
  South_Outer_concrete_wall_temperature_[K]/1 -> Mux1/2
  Mux2/1 -> "(1/R)=1/{L/(kA)_concrete+L/(kA)_insulator}1"/1
  Gain3/1 -> Mux2/4
  [OuterWall_Depth] -> Gain2/1
  [Ambient_Temp_K] -> T/2

== system building_HVAC_V00_027_AI_2019b/Building_Block/West_Wall_Block/Subsystem1 ==
  West_inner_concrete_wall_temperature_[K] : Inport
  Inner_air_temperature_[K] : Inport  Port=2
  West_Inner_Convective_coefficient_h : Inport  Port=3
  -1000000 to 1000000 : Saturate  UpperLimit=1000000  LowerLimit=-1000000
  Memory : Memory  InheritSampleTime=on
  Mux4 : Mux
  Q=hA(dT) : Fcn  Expr=u(1)*u(2)*(u(3)-u(4))
  Q_West_InnerWall_to_InnerAir_[W] : Outport
  wires:
  West_Inner_Convective_coefficient_h/1 -> Mux4/1
  [Area_West] -> Mux4/2
  West_inner_concrete_wall_temperature_[K]/1 -> Mux4/3
  -1000000 to 1000000/1 -> Q_West_InnerWall_to_InnerAir_[W]/1
  Mux4/1 -> Q=hA(dT)/1
  Q=hA(dT)/1 -> Memory/1
  Memory/1 -> -1000000 to 1000000/1
  Inner_air_temperature_[K]/1 -> Mux4/4

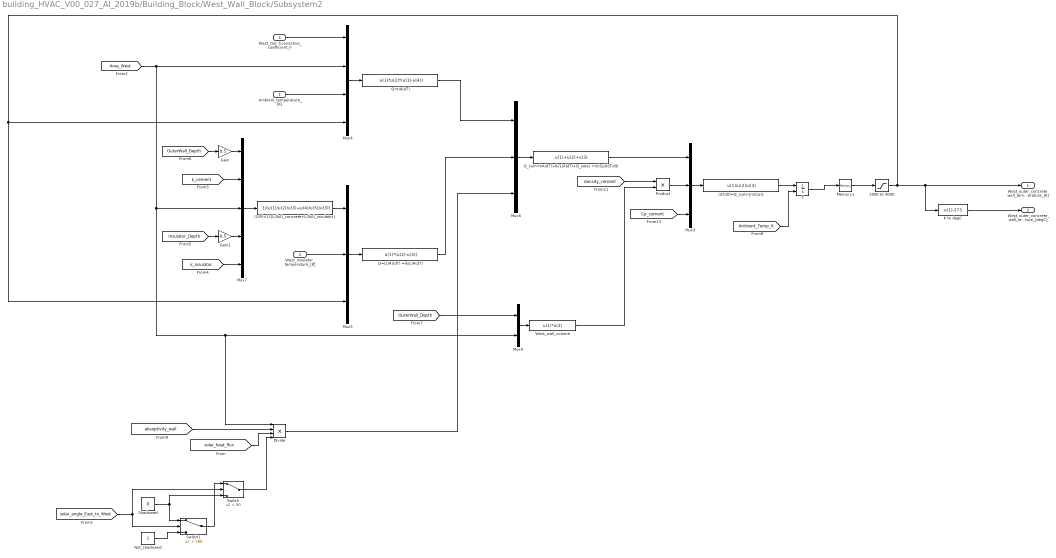
== system building_HVAC_V00_027_AI_2019b/Building_Block/West_Wall_Block/Subsystem2 ==
  Ambient_temperature_[K] : Inport
  West_Insulator_temperature_[K] : Inport  Port=2
  West_Out_Convective_coefficient_h : Inport  Port=3
  "(1/R)=1/{L/(kA)_concrete+L/(kA)_insulator}" : Fcn  Expr=1/(u(1)/u(2)/u(3)+u(4)/u(5)/u(3))
  "(dT/dt)=Q_sum/{m(Cp)}" : Fcn  Expr=u(1)/u(2)/u(3)
  200K to 400K : Saturate  UpperLimit=400  LowerLimit=200
  Divide : Product  Inputs=****
  Gain : Gain  Gain=0.5
  Gain1 : Gain  Gain=0.5
  K to degC : Fcn  Expr=u(1)-273
  Memory1 : Memory  InitialCondition=300  InheritSampleTime=on
  Mux3 : Mux  Inputs=3
  Mux4 : Mux
  Mux5 : Mux  Inputs=3
  Mux6 : Mux  Inputs=3
  Mux7 : Mux  Inputs=5
  Mux9 : Mux  Inputs=2
  Not_shadowed : Constant
  Product : Product
  Q=(1/R)(dT) =(k/L)A(dT) : Fcn  Expr=u(1)*(u(2)-u(3))
  Q=hA(dT) : Fcn  Expr=u(1)*u(2)*(u(3)-u(4))
  Q_sum=hA(dT)+(k/L)A(dT)+Q_solar =m(Cp)(dT/dt) : Fcn  Expr=u(1)+u(2)+u(3)
  Shadowed : Constant  Value=0
  Switch : Switch  Criteria=u2 > Threshold  Threshold=90
  Switch1 : Switch  Criteria=u2 > Threshold  Threshold=180
  T : Integrator  InitialConditionSource=external
  West_wall_volume : Fcn  Expr=u(1)*u(2)
  West_outer_concrete_wall_temperature_[K] : Outport
  West_outer_concrete_wall_temperature_[degC] : Outport  Port=2
  wires:
  Switch/1 -> Divide/4
  Shadowed/1 -> Switch1/1, Switch/3
  Not_shadowed/1 -> Switch1/3
  Switch1/1 -> Switch/1
  [solar_angle_East_to_West] -> Switch1/2, Switch/2
  Mux6/1 -> Q_sum=hA(dT)+(k/L)A(dT)+Q_solar =m(Cp)(dT/dt)/1
  West_Out_Convective_coefficient_h/1 -> Mux4/1
  Mux3/1 -> "(dT/dt)=Q_sum/{m(Cp)}"/1
  [density_cement] -> Product/1
  Mux9/1 -> West_wall_volume/1
  "(dT/dt)=Q_sum/{m(Cp)}"/1 -> T/1
  [Cp_cement] -> Mux3/3
  Product/1 -> Mux3/2
  [OuterWall_Depth] -> Mux9/1
  Ambient_temperature_[K]/1 -> Mux4/3
  [OuterWall_Depth] -> Gain/1
  T/1 -> Memory1/1
  200K to 400K/1 -> K to degC/1, West_outer_concrete_wall_temperature_[K]/1, Mux4/4, Mux5/3
  Mux5/1 -> Q=(1/R)(dT) =(k/L)A(dT)/1
  Mux4/1 -> Q=hA(dT)/1
  Q=(1/R)(dT) =(k/L)A(dT)/1 -> Mux6/2
  Memory1/1 -> 200K to 400K/1
  [Insulator_Depth] -> Gain1/1
  Gain/1 -> Mux7/1
  "(1/R)=1/{L/(kA)_concrete+L/(kA)_insulator}"/1 -> Mux5/1
  Q=hA(dT)/1 -> Mux6/1
  Mux7/1 -> "(1/R)=1/{L/(kA)_concrete+L/(kA)_insulator}"/1
  [k_cement] -> Mux7/2
  Q_sum=hA(dT)+(k/L)A(dT)+Q_solar =m(Cp)(dT/dt)/1 -> Mux3/1
  West_Insulator_temperature_[K]/1 -> Mux5/2
  Gain1/1 -> Mux7/4
  [k_insulator] -> Mux7/5
  West_wall_volume/1 -> Product/2
  K to degC/1 -> West_outer_concrete_wall_temperature_[degC]/1
  [Area_West] -> Mux9/2, Divide/1, Mux7/3, Mux4/2
  Divide/1 -> Mux6/3
  [solar_heat_flux] -> Divide/3
  [absoptivity_wall] -> Divide/2
  [Ambient_Temp_K] -> T/2

== system building_HVAC_V00_027_AI_2019b/Building_Block/West_Wall_Block/Subsystem3 ==
  West_Insulator_temperature_[K] : Inport
  Inner_air_temperature_[K] : Inport  Port=2
  West_Inner_Convective_coefficient_h : Inport  Port=3
  "(1/R)=1/{L/(kA)_concrete+L/(kA)_insulator}" : Fcn  Expr=1/(u(1)/u(2)/u(3)+u(4)/u(5)/u(3))
  "(dT/dt)=Q_sum/{m(Cp)}" : Fcn  Expr=u(1)/u(2)/u(3)
  200K to 400K : Saturate  UpperLimit=400  LowerLimit=200
  Divide : Product  Inputs=**
  Gain : Gain  Gain=0.5
  Gain1 : Gain  Gain=0.5
  K to degC : Fcn  Expr=u(1)-273
  Memory1 : Memory  InitialCondition=300  InheritSampleTime=on
  Mux3 : Mux  Inputs=3
  Mux4 : Mux
  Mux5 : Mux  Inputs=3
  Mux6 : Mux  Inputs=3
  Mux7 : Mux  Inputs=5
  Mux9 : Mux  Inputs=2
  Product : Product
  Q=(1/R)(dT) =(k/L)A(dT) : Fcn  Expr=u(1)*(u(2)-u(3))
  Q=hA(dT) : Fcn  Expr=u(1)*u(2)*(u(3)-u(4))
  Q_sum=hA(dT)+(k/L)A(dT)+Q_solar =m(Cp)(dT/dt) : Fcn  Expr=u(1)+u(2)
  T : Integrator  InitialConditionSource=external
  West_wall_volume : Fcn  Expr=u(1)*u(2)
  West_inner_concrete_wall_temperature_[K] : Outport
  West_inner_concrete_wall_temperature_[degC] : Outport  Port=2
  wires:
  K to degC/1 -> West_inner_concrete_wall_temperature_[degC]/1
  West_wall_volume/1 -> Product/2
  [k_insulator] -> Mux7/5
  Gain1/1 -> Mux7/4
  West_Insulator_temperature_[K]/1 -> Mux5/2
  Q_sum=hA(dT)+(k/L)A(dT)+Q_solar =m(Cp)(dT/dt)/1 -> Mux3/1
  [k_cement] -> Mux7/2
  Mux7/1 -> "(1/R)=1/{L/(kA)_concrete+L/(kA)_insulator}"/1
  Q=hA(dT)/1 -> Mux6/1
  "(1/R)=1/{L/(kA)_concrete+L/(kA)_insulator}"/1 -> Mux5/1
  Gain/1 -> Mux7/1
  [Insulator_Depth] -> Gain1/1
  Memory1/1 -> 200K to 400K/1
  Q=(1/R)(dT) =(k/L)A(dT)/1 -> Mux6/2
  Mux4/1 -> Q=hA(dT)/1
  Mux5/1 -> Q=(1/R)(dT) =(k/L)A(dT)/1
  200K to 400K/1 -> Mux5/3, Mux4/4, West_inner_concrete_wall_temperature_[K]/1, K to degC/1
  T/1 -> Memory1/1
  [InnerWall_Depth] -> Gain/1
  Inner_air_temperature_[K]/1 -> Mux4/3
  [Area_West] -> Mux9/2, Mux7/3, Mux4/2
  [InnerWall_Depth] -> Mux9/1
  Product/1 -> Mux3/2
  [Cp_cement] -> Mux3/3
  "(dT/dt)=Q_sum/{m(Cp)}"/1 -> T/1
  Mux9/1 -> West_wall_volume/1
  [density_cement] -> Product/1
  Mux3/1 -> "(dT/dt)=Q_sum/{m(Cp)}"/1
  West_Inner_Convective_coefficient_h/1 -> Mux4/1
  Mux6/1 -> Q_sum=hA(dT)+(k/L)A(dT)+Q_solar =m(Cp)(dT/dt)/1
  [Ambient_Temp_K] -> T/2
  [absorptivity_inner_wall_West] -> Divide/2
  [Q_solar_to_InnerAir] -> Divide/1
  Divide/1 -> Mux6/3

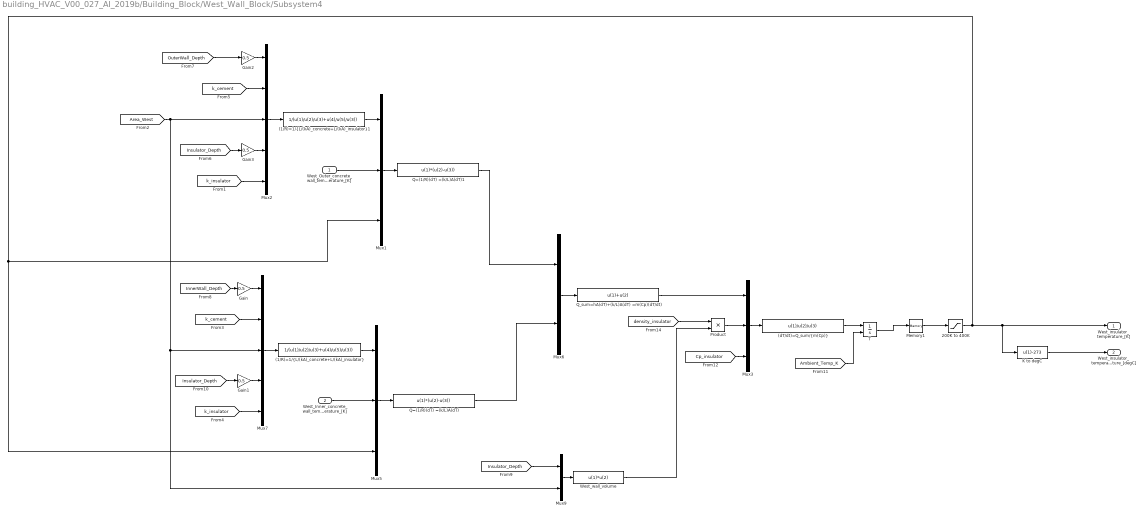
== system building_HVAC_V00_027_AI_2019b/Building_Block/West_Wall_Block/Subsystem4 ==
  West_Outer_concrete_wall_temperature_[K] : Inport
  West_Inner_concrete_wall_temperature_[K] : Inport  Port=2
  "(1/R)=1/{L/(kA)_concrete+L/(kA)_insulator}" : Fcn  Expr=1/(u(1)/u(2)/u(3)+u(4)/u(5)/u(3))
  "(1/R)=1/{L/(kA)_concrete+L/(kA)_insulator}1" : Fcn  Expr=1/(u(1)/u(2)/u(3)+u(4)/u(5)/u(3))
  "(dT/dt)=Q_sum/{m(Cp)}" : Fcn  Expr=u(1)/u(2)/u(3)
  200K to 400K : Saturate  UpperLimit=400  LowerLimit=200
  Gain{,1..3} (4 alike) : Gain  Gain=0.5
  K to degC : Fcn  Expr=u(1)-273
  Memory1 : Memory  InitialCondition=300  InheritSampleTime=on
  Mux1 : Mux  Inputs=3
  Mux2 : Mux  Inputs=5
  Mux3 : Mux  Inputs=3
  Mux5 : Mux  Inputs=3
  Mux6 : Mux  Inputs=2
  Mux7 : Mux  Inputs=5
  Mux9 : Mux  Inputs=2
  Product : Product
  Q=(1/R)(dT) =(k/L)A(dT) : Fcn  Expr=u(1)*(u(2)-u(3))
  Q=(1/R)(dT) =(k/L)A(dT)1 : Fcn  Expr=u(1)*(u(2)-u(3))
  Q_sum=hA(dT)+(k/L)A(dT) =m(Cp)(dT/dt) : Fcn  Expr=u(1)+u(2)
  T : Integrator  InitialConditionSource=external
  West_wall_volume : Fcn  Expr=u(1)*u(2)
  West_insulator_temperature_[K] : Outport
  West_insulator_temperature_[degC] : Outport  Port=2
  wires:
  Mux6/1 -> Q_sum=hA(dT)+(k/L)A(dT) =m(Cp)(dT/dt)/1
  Mux3/1 -> "(dT/dt)=Q_sum/{m(Cp)}"/1
  [density_insulator] -> Product/1
  Mux9/1 -> West_wall_volume/1
  "(dT/dt)=Q_sum/{m(Cp)}"/1 -> T/1
  [Cp_insulator] -> Mux3/3
  Product/1 -> Mux3/2
  [Insulator_Depth] -> Mux9/1
  [Area_West] -> Mux9/2, Mux7/3, Mux2/3
  [InnerWall_Depth] -> Gain/1
  T/1 -> Memory1/1
  200K to 400K/1 -> K to degC/1, West_insulator_temperature_[K]/1, Mux1/3, Mux5/3
  Mux5/1 -> Q=(1/R)(dT) =(k/L)A(dT)/1
  Q=(1/R)(dT) =(k/L)A(dT)/1 -> Mux6/2
  Memory1/1 -> 200K to 400K/1
  [Insulator_Depth] -> Gain1/1
  Gain/1 -> Mux7/1
  "(1/R)=1/{L/(kA)_concrete+L/(kA)_insulator}"/1 -> Mux5/1
  Q=(1/R)(dT) =(k/L)A(dT)1/1 -> Mux6/1
  Mux7/1 -> "(1/R)=1/{L/(kA)_concrete+L/(kA)_insulator}"/1
  [k_cement] -> Mux7/2
  Q_sum=hA(dT)+(k/L)A(dT) =m(Cp)(dT/dt)/1 -> Mux3/1
  West_Inner_concrete_wall_temperature_[K]/1 -> Mux5/2
  Gain1/1 -> Mux7/4
  [k_insulator] -> Mux7/5
  West_wall_volume/1 -> Product/2
  K to degC/1 -> West_insulator_temperature_[degC]/1
  [k_insulator] -> Mux2/5
  "(1/R)=1/{L/(kA)_concrete+L/(kA)_insulator}1"/1 -> Mux1/1
  Gain2/1 -> Mux2/1
  [k_cement] -> Mux2/2
  [Insulator_Depth] -> Gain3/1
  Mux1/1 -> Q=(1/R)(dT) =(k/L)A(dT)1/1
  West_Outer_concrete_wall_temperature_[K]/1 -> Mux1/2
  Mux2/1 -> "(1/R)=1/{L/(kA)_concrete+L/(kA)_insulator}1"/1
  Gain3/1 -> Mux2/4
  [OuterWall_Depth] -> Gain2/1
  [Ambient_Temp_K] -> T/2

== system building_HVAC_V00_027_AI_2019b/Building_Block/Blower_and_InnerAir_Block/Mass_H2O_vapor_InnerAir/Subsystem ==
  Ambient_temperature_[K]2 : Inport
  Mux12 : Mux
  m=PV/RT : Fcn  Expr=u(1)*u(2)/u(3)/u(4)
  Out1 : Outport
  wires:
  [Volume_room] -> Mux12/2
  Mux12/1 -> m=PV/RT/1
  [gas_constant_water] -> Mux12/3
  Ambient_temperature_[K]2/1 -> Mux12/4
  [pressure_H2O_vapor] -> Mux12/1
  m=PV/RT/1 -> Out1/1

== system building_HVAC_V00_027_AI_2019b/Building_Block/Blower_and_InnerAir_Block/Mass_dry_air_InnerAir/Subsystem1 ==
  Ambient_temperature_[K]2 : Inport
  Mux12 : Mux
  m=PV/RT : Fcn  Expr=u(1)*u(2)/u(3)/u(4)
  Out1 : Outport
  wires:
  m=PV/RT/1 -> Out1/1
  [atmosphere_pressure] -> Mux12/1
  Ambient_temperature_[K]2/1 -> Mux12/4
  [gas_constant_dry_air] -> Mux12/3
  Mux12/1 -> m=PV/RT/1
  [Volume_room] -> Mux12/2

== matlab function building_HVAC_V00_027_AI_2019b/MATLAB Function1 ==
  data: temp input; out output; dtemp input; power input; preout input; c_t input; energy input; next_t input; n_t output; s_time input; outtemp input; outdtemp input
% function [out, n_t] = ActionLogic(temp,dtemp,power,preout,c_t, energy, next_t, s_time)
%     data = 0;
%    out = preout;
%    n_t = next_t;
%     token = mod(c_t, next_t);
%     if token ~= 0 || c_t == 0
%         out = preout;
%         n_t = next_t; 
%     else
%        data = usePython(temp, dtemp, power, energy, c_t);
%         if data < 0
%             out = 0;
%             n_t = s_time - data;
%         else
%             out = 1;
%             n_t = s_time + data;
%         end
%     end
% end
function [out, n_t] = ActionLogic(temp,dtemp,power,preout,c_t, energy, next_t, s_time, outtemp, outdtemp)
    data = 0;
%    out = preout;
%    n_t = next_t;
    token = mod(c_t, next_t);
    if token ~= 0 || c_t == 0
        out = preout;
        n_t = next_t; 
    else
        data = usePython(temp, dtemp, power, energy, c_t, outtemp, outdtemp);
        if data < 0
            out = 0;
            n_t = s_time - data;
        else
            out = 1;
            n_t = s_time + data;
        end
    end
end

== matlab function building_HVAC_V00_027_AI_2019b/MATLAB Function2 ==
  data: temp input; out output; dtemp input; power input; preout input; c_t input; energy input; next_t input; n_t output; s_time input; outtemp input; outdtemp input
function [out, n_t] = ActionLogic(temp,dtemp,power,preout,c_t, energy, next_t, s_time, outtemp, outdtemp)
    out = 1;
    n_t = 0;
end
